simulink model "Week2_prob1"  (R2020b)
settings: Solver=VariableStepAuto  StartTime=0.0  StopTime=10.0  RelTol=1e-3
settings Model: Creator=Lakshmi  LastModifiedBy=Lakshmi

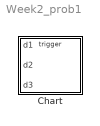
== system Week2_prob1 ==
  Chart : Stateflow chart  TreatAsAtomicUnit=on

== stateflow chart Week2_prob1/Chart ==
  settings: executeAtInitialization=1
  state Digit1
    state one
      en:d1=1;
    state zero
      en:d1=0;
    state two
      en:d1=2;
    state four
      en:d1=4;
    state three
      en:d1=3;
    (default) -> Digit1.zero
    Digit1.zero -> Digit1.one
    Digit1.one -> Digit1.two
    Digit1.two -> Digit1.three
    Digit1.three -> Digit1.four
    Digit1.four -> Digit1.zero
  state Digit2
    state one
      en:d2=1;
    state zero
      en:d2=0;
    state two
      en:d2=2;
    state four
      en:d2=4;
    state three
      en:d2=3;
    (default) -> Digit2.zero
    Digit2.zero -> Digit2.one
    Digit2.one -> Digit2.two
    Digit2.two -> Digit2.three
    Digit2.three -> Digit2.four
    Digit2.four -> Digit2.zero
  state Digit3
    state one
      en:d3=1;
    state zero
      en:d3=0;
    state two
      en:d3=2;
    state four
      en:d3=4;
    state three
      en:d3=3;
    (default) -> Digit3.zero
    Digit3.zero -> Digit3.one
    Digit3.one -> Digit3.two
    Digit3.two -> Digit3.three
    Digit3.three -> Digit3.four
    Digit3.four -> Digit3.zero
  data: d1 input; d2 input; d3 input
  events: inc2 local FUNCTION_CALL_EVENT; inc3 local FUNCTION_CALL_EVENT; InputClick input FUNCTION_CALL_EVENT
